simulink model "buck_hvoltage2_org"  (Simulink 10.0)
settings: Solver=ode45  StartTime=0.0  StopTime=Tmax  RelTol=1e-3  EnableMultiTasking=on
undefined symbols (not defined in the file): a00c, a00d, a00o, a01c, a01d, a01o, a10c, a10d, a10o, a11c, a11d, a11o, b0c, b0d, b0o, b1c, b1d, b1o, D, i0, T, v0, Vref, Vs, Vs_noise, Vtol
settings Model: Creator=Omar Ali Beg  LastModifiedBy=annonymous
settings DataIOCC: LimitDataPoints=on  SignalLoggingSaveFormat=ModelDataLogs
settings OptimizationCC: ExpressionDepthLimit=2147483647
settings DebuggingCC: MaxConsecutiveZCsMsg=none  SolverPrmCheckMsg=warning  MultiTaskDSMMsg=warning  MultiTaskCondExecSysMsg=none  StateNameClashWarn=warning
settings GRTTargetCC: GeneratePreprocessorConditionals=Disable all  CombineOutputUpdateFcns=on  GRTInterface=off
settings ConfigComp: CovExternalEMLEnable=off

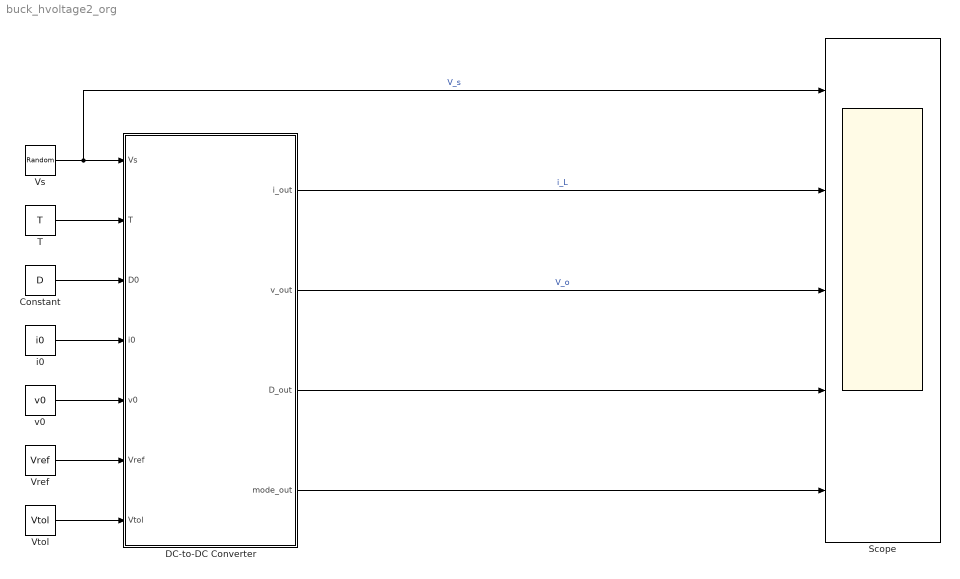
== system buck_hvoltage2_org ==
  Constant : Constant  Value=D
  DC-to-DC Converter : Stateflow chart  TreatAsAtomicUnit=on
  Scope : Scope  NumInputPorts=5
  T : Constant  Value=T
  Vref : Constant  Value=Vref
  Vs : RandomNumber  Mean=Vs  Variance=Vs_noise  SampleTime=T/10
  Vtol : Constant  Value=Vtol
  i0 : Constant  Value=i0
  v0 : Constant  Value=v0
  wires:
  DC-to-DC Converter/1(i_out) -> Scope/2  "i_L"
  DC-to-DC Converter/2(v_out) -> Scope/3  "V_o"
  T/1 -> DC-to-DC Converter/2(T)
  Vs/1 -> Scope/1, DC-to-DC Converter/1(Vs)  "V_s"
  i0/1 -> DC-to-DC Converter/4(i0)
  v0/1 -> DC-to-DC Converter/5(v0)
  Constant/1 -> DC-to-DC Converter/3(D0)
  Vref/1 -> DC-to-DC Converter/6(Vref)
  DC-to-DC Converter/3(D_out) -> Scope/4
  DC-to-DC Converter/4(mode_out) -> Scope/5
  Vtol/1 -> DC-to-DC Converter/7(Vtol)

== stateflow chart DC-to-DC Converter ==
  settings: updateMethod=CONTINUOUS
  state Discontinuous
    du:
    i_dot = a00d*i+a01d*v+b0d*Vs;
    v_dot = a10d*i+a11d*v+b1d*Vs;
    t_dot = 1;
    i_out =i;
    v_out = v;
    D_out=D;
    mode_out=3;
  state Charging
    du:
    i_dot = a00c*i+a01c*v+b0c*Vs;
    v_dot = a10c*i+a11c*v+b1c*Vs;
    t_dot = 1;
    i_out = i;
    v_out = v;
    D_out=D;
    mode_out=2;
  state Discharging
    du:
    i_dot = a00o*i+a01o*v+b0o*Vs;
    v_dot = a10o*i+a11o*v+b1o*Vs;
    t_dot = 1;
    i_out = i;
    v_out = v;
    D_out=D;
    mode_out=1;
  Discharging -> Discontinuous [order 1] : [i <= 0]
  Discontinuous -> Charging : [v <= Vref-Vtol]
  Charging -> Discharging : [v >= Vref+Vtol]
  Discharging -> Charging [order 2] : [v <= Vref-Vtol]
  (default) -> Charging : {i = i0;
      | v = v0;
      | D=D;}
  data: t local double; i_out output double; v_out output double; i local double; a00o local double =a00o; Vs input double =120; T input double; D0 input double =D0; a01o local double =a01o; a10o local double =a10o; a11o local double =a11o; a00c local double =a00c; a01c local double =a01c; a10c local double =a10c; a11c local double =a11c; b0o local double =b0o; b1o local double =b1o; b0c local double =b0c; b1c local double =b1c; v local double; i0 input double; v0 input double; a01d local double =a01d; a10d local double =a10d; a11d local double =a11d; a00d local double =a00d; b0d local double =b0d; b1d local double =b1d; Vref input double =120; D local double; v1 local double; D_out output double; mode_out output double; Vtol input double =120
  data t settings: updateMethod=SF_CONTINUOUS_TIME_DATA
  data i settings: updateMethod=SF_CONTINUOUS_TIME_DATA
  data v settings: updateMethod=SF_CONTINUOUS_TIME_DATA
  data D settings: updateMethod=SF_CONTINUOUS_TIME_DATA
  data v1 settings: updateMethod=SF_CONTINUOUS_TIME_DATA
  data Vtol settings: description=Voltage tolerance (e.g., Vref / 100 is +/- 1% voltage ripple)
